simulink model "lab9p1"  (R2015a)
settings: Solver=ode45  StartTime=0.0  StopTime=20.0  RelTol=1e-3
libraries: simulink x2
settings Model: Creator=dg  LastModifiedBy=dg

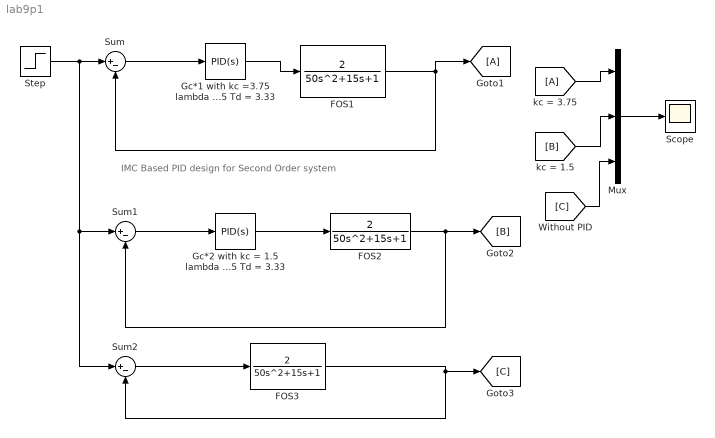
== system lab9p1 ==
  note: IMC Based PID design for Second Order system
  " Gc*1 with kc =3.75 lambda = 2 Ti = 15 Td = 3.33" : simulink/Continuous/PID Controller  Controller=PID  TimeDomain=Continuous-time  SampleTime=-1  IntegratorMethod=Forward Euler  FilterMethod=Forward Euler  Form=Ideal  UseFilter=on  ControllerParametersSource=internal  P=3.75  I=1/15  D=3.33  N=100  InitialConditionSource=internal  InitialConditionForIntegrator=0  InitialConditionForFilter=0  ExternalReset=none  LimitOutput=off  UpperSaturationLimit=inf  LowerSaturationLimit=-inf  LinearizeAsGain=on  AntiWindupMode=none  Kb=1  TrackingMode=off  Kt=1  PParamMin=[]  PParamMax=[]  IParamMin=[]  IParamMax=[]  DParamMin=[]  DParamMax=[]  NParamMin=[]  NParamMax=[]  KbParamMin=[]  KbParamMax=[]  KtParamMin=[]  KtParamMax=[]  POutMin=[]  POutMax=[]  IOutMin=[]  IOutMax=[]  DOutMin=[]  DOutMax=[]  NOutMin=[]  NOutMax=[]  KbOutMin=[]  KbOutMax=[]  KtOutMin=[]  KtOutMax=[]  IntegratorOutMin=[]  IntegratorOutMax=[]  FilterOutMin=[]  FilterOutMax=[]  SumOutMin=[]  SumOutMax=[]  SumI1OutMin=[]  SumI1OutMax=[]  SumI2OutMin=[]  SumI2OutMax=[]  SumI3OutMin=[]  SumI3OutMax=[]  SumDOutMin=[]  SumDOutMax=[]  SaturationOutMin=[]  SaturationOutMax=[]  IntegratorContinuousStateAttributes=''  IntegratorStateMustResolveToSignalObject=off  IntegratorRTWStateStorageClass=Auto  FilterContinuousStateAttributes=''  FilterStateMustResolveToSignalObject=off  FilterRTWStateStorageClass=Auto  DifferentiatorICPrevScaledInput=0  DifferentiatorOutMin=[]  DifferentiatorOutMax=[]
  " Gc*2 with kc = 1.5 lambda = 5 Ti = 15 Td = 3.33" : simulink/Continuous/PID Controller  Controller=PID  TimeDomain=Continuous-time  SampleTime=-1  IntegratorMethod=Forward Euler  FilterMethod=Forward Euler  Form=Ideal  UseFilter=on  ControllerParametersSource=internal  P=1.5  I=1/15  D=3.33  N=100  InitialConditionSource=internal  InitialConditionForIntegrator=0  InitialConditionForFilter=0  ExternalReset=none  LimitOutput=off  UpperSaturationLimit=inf  LowerSaturationLimit=-inf  LinearizeAsGain=on  AntiWindupMode=none  Kb=1  TrackingMode=off  Kt=1  PParamMin=[]  PParamMax=[]  IParamMin=[]  IParamMax=[]  DParamMin=[]  DParamMax=[]  NParamMin=[]  NParamMax=[]  KbParamMin=[]  KbParamMax=[]  KtParamMin=[]  KtParamMax=[]  POutMin=[]  POutMax=[]  IOutMin=[]  IOutMax=[]  DOutMin=[]  DOutMax=[]  NOutMin=[]  NOutMax=[]  KbOutMin=[]  KbOutMax=[]  KtOutMin=[]  KtOutMax=[]  IntegratorOutMin=[]  IntegratorOutMax=[]  FilterOutMin=[]  FilterOutMax=[]  SumOutMin=[]  SumOutMax=[]  SumI1OutMin=[]  SumI1OutMax=[]  SumI2OutMin=[]  SumI2OutMax=[]  SumI3OutMin=[]  SumI3OutMax=[]  SumDOutMin=[]  SumDOutMax=[]  SaturationOutMin=[]  SaturationOutMax=[]  IntegratorContinuousStateAttributes=''  IntegratorStateMustResolveToSignalObject=off  IntegratorRTWStateStorageClass=Auto  FilterContinuousStateAttributes=''  FilterStateMustResolveToSignalObject=off  FilterRTWStateStorageClass=Auto  DifferentiatorICPrevScaledInput=0  DifferentiatorOutMin=[]  DifferentiatorOutMax=[]
  FOS1 : TransferFcn  Numerator=[2]  Denominator=[50 15 1]
  FOS2 : TransferFcn  Numerator=[2]  Denominator=[50 15 1]
  FOS3 : TransferFcn  Numerator=[2]  Denominator=[50 15 1]
  Mux : Mux  Inputs=3
  Scope : Scope
      settings: ShowLegends=on  SampleInput=on
  Step : Step  SampleTime=0
  Sum : Sum  Inputs=|+-
  Sum1 : Sum  Inputs=|+-
  Sum2 : Sum  Inputs=|+-
  wires:
  FOS1/1 -> [A], Sum/2
  " Gc*1 with kc =3.75 lambda = 2 Ti = 15 Td = 3.33"/1 -> FOS1/1
  Sum/1 -> " Gc*1 with kc =3.75 lambda = 2 Ti = 15 Td = 3.33"/1
  [A] -> Mux/1
  [B] -> Mux/2
  Mux/1 -> Scope/1
  FOS2/1 -> [B], Sum1/2
  " Gc*2 with kc = 1.5 lambda = 5 Ti = 15 Td = 3.33"/1 -> FOS2/1
  Sum1/1 -> " Gc*2 with kc = 1.5 lambda = 5 Ti = 15 Td = 3.33"/1
  FOS3/1 -> [C], Sum2/2
  Sum2/1 -> FOS3/1
  Step/1 -> Sum2/1, Sum1/1, Sum/1
  [C] -> Mux/3
